simulink model "linmodel_eq1_discr3"  (R2019a)
settings: Solver=VariableStepAuto  StartTime=0.0  StopTime=30  RelTol=1e-3
InitFcn:
  | lin_discr_model
undefined symbols (not defined in the file): A_eq1_d2, B_eq1_d2, C_eq1_d2, L2, Ts
settings Model: Creator=jessi  LastModifiedBy=jessi

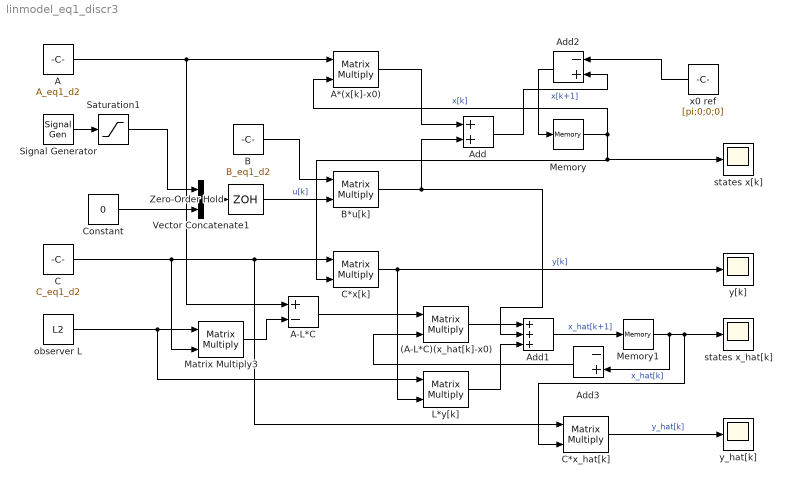
== system linmodel_eq1_discr3 ==
  (A-L*C)(x_hat[k]-x0) : Product  Multiplication=Matrix(*)
  A : Constant  Value=A_eq1_d2  SampleTime=Ts
  A*(x[k]-x0) : Product  Multiplication=Matrix(*)
  A-L*C : Sum  Inputs=+-
  Add : Sum
  Add1 : Sum  Inputs=+++
  Add2 : Sum  Inputs=-+
  Add3 : Sum  Inputs=-+
  B : Constant  Value=B_eq1_d2  SampleTime=Ts
  B*u[k] : Product  Multiplication=Matrix(*)
  C : Constant  Value=C_eq1_d2  SampleTime=Ts
  C*x[k] : Product  Multiplication=Matrix(*)
  C*x_hat[k] : Product  Multiplication=Matrix(*)
  Constant : Constant  Value=0
  L*y[k] : Product  Multiplication=Matrix(*)
  Matrix Multiply3 : Product  Multiplication=Matrix(*)
  Memory : Memory  InitialCondition=[pi;0;0;0]
  Memory1 : Memory  InitialCondition=[pi;0;0;0]
  Saturation1 : Saturate  UpperLimit=1  LowerLimit=-1
  Signal Generator : SignalGenerator  WaveForm=square  Amplitude=-0.3
  Vector Concatenate1 : Concatenate
  Zero-Order Hold : ZeroOrderHold  SampleTime=Ts
  observer L : Constant  Value=L2  SampleTime=Ts
  states x[k] : Scope
  states x_hat[k] : Scope
  x0 ref : Constant  Value=[pi;0;0;0]  SampleTime=Ts
  y[k] : Scope
  y_hat[k] : Scope
  wires:
  Constant/1 -> Vector Concatenate1/2
  Signal Generator/1 -> Saturation1/1
  Saturation1/1 -> Vector Concatenate1/1
  Vector Concatenate1/1 -> Zero-Order Hold/1
  Zero-Order Hold/1 -> B*u[k]/2  "u[k]"
  B/1 -> B*u[k]/1
  A/1 -> A-L*C/1, A*(x[k]-x0)/1
  A*(x[k]-x0)/1 -> Add/1
  B*u[k]/1 -> Add1/2, Add/2
  Memory/1 -> A*(x[k]-x0)/2, states x[k]/1, C*x[k]/2  "x[k]"
  C/1 -> Matrix Multiply3/2, C*x_hat[k]/1, C*x[k]/1
  C*x[k]/1 -> L*y[k]/2, y[k]/1  "y[k]"
  observer L/1 -> L*y[k]/1, Matrix Multiply3/1
  Matrix Multiply3/1 -> A-L*C/2
  A-L*C/1 -> (A-L*C)(x_hat[k]-x0)/1
  (A-L*C)(x_hat[k]-x0)/1 -> Add1/1
  L*y[k]/1 -> Add1/3
  Add1/1 -> Memory1/1  "x_hat[k+1]"
  Memory1/1 -> Add3/2, C*x_hat[k]/2, states x_hat[k]/1  "x_hat[k]"
  C*x_hat[k]/1 -> y_hat[k]/1  "y_hat[k]"
  x0 ref/1 -> Add2/1
  Add3/1 -> (A-L*C)(x_hat[k]-x0)/2
  Add/1 -> Add2/2  "x[k+1]"
  Add2/1 -> Memory/1
